simulink library "tinbot"  (R2016a)
settings: Solver=ode45  StartTime=0.0  StopTime=10.0  RelTol=1e-3
libraries: tinbot x23, simulink x4
settings Model: Creator=maximilian  LastModifiedBy=maximilian
settings DataIOCC: LimitDataPoints=on
settings DebuggingCC: AllowSymbolicDim=off

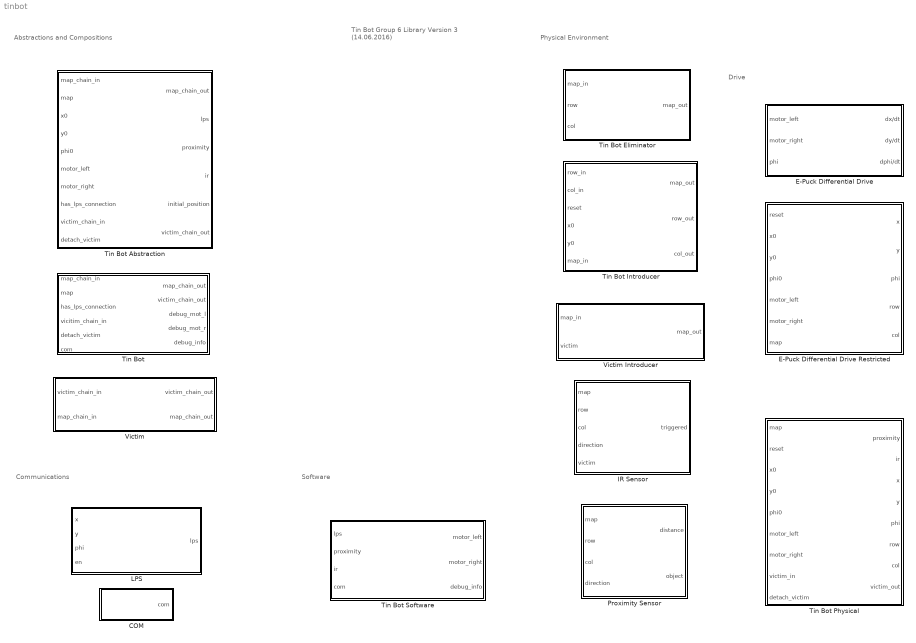
== system tinbot ==
  note: Abstractions and Compositions
  note: Tin Bot
      | Group 6
      |
      | Library
      | Version 3
      | (14.06.2016)
  note: Communications
  note: Physical Environment
  note: Software
  note: Drive
  COM : Subsystem
      mask Display: fprintf('COM')
  E-Puck Differential Drive : Subsystem  TreatAsAtomicUnit=on
      mask Display: fprintf('E-Puck\nDifferential Drive')
  E-Puck Differential Drive Restricted : Subsystem
      mask Display: fprintf('E-Puck\nDifferential Drive\n(restricted)')
  IR Sensor : Subsystem
      mask Display: fprintf('IR Sensor')
  LPS : Subsystem
      mask Display: fprintf('LPS')
  Proximity Sensor : Subsystem
      mask Display: fprintf('Proximity Sensor')
  Tin Bot : Subsystem  mask{x0=100, y0=100, phi0=0}
      mask Display: fprintf('Tin Bot')
  Tin Bot Abstraction : Subsystem
      mask Display: fprintf('Tin Bot\n(abstract)')
  Tin Bot Eliminator : Subsystem
      mask Display: fprintf('Tin Bot\nEliminator')
  Tin Bot Introducer : Subsystem
      mask Display: fprintf('Tin Bot\nIntroducer')
  Tin Bot Physical : Subsystem
      mask Display: fprintf('Tin Bot\nPhysical\n(with motor delay)')
  Tin Bot Software : Subsystem
      mask Display: fprintf('Tin Bot\nSoftware');
  Victim : Subsystem  mask{x0=100, y0=100}
      mask Display: fprintf('Victim')
  Victim Introducer : Subsystem
      mask Display: fprintf('Victim\nIntroducer')

== system tinbot/COM ==
  Chart : Stateflow chart
  com : Outport
  wires:
  Chart/1(com) -> com/1

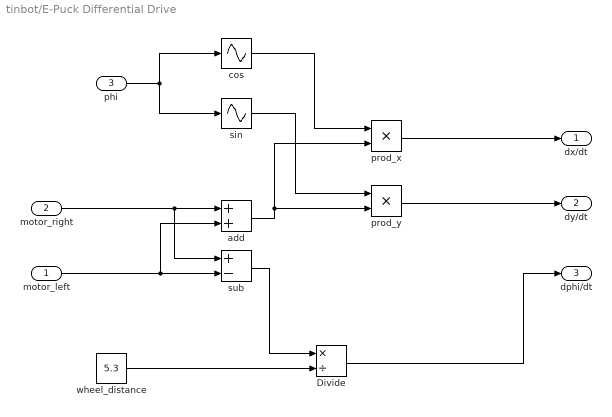
== system tinbot/E-Puck Differential Drive ==
  motor_left : Inport
  motor_right : Inport  Port=2
  phi : Inport  Port=3
  Divide : Product  Inputs=*/
  add : Sum
  cos : Sin  TimeSource=Use external signal  Amplitude=0.5  Phase=pi/2  SampleTime=0
  prod_x : Product
  prod_y : Product
  "sin " : Sin  TimeSource=Use external signal  Amplitude=0.5  SampleTime=0
  sub : Sum  Inputs=+-
  wheel_distance : Constant  Value=5.3
  dx/dt : Outport
  dy/dt : Outport  Port=2
  dphi/dt : Outport  Port=3
  wires:
  motor_left/1 -> sub/2, add/2
  motor_right/1 -> sub/1, add/1
  sub/1 -> Divide/1
  wheel_distance/1 -> Divide/2
  Divide/1 -> dphi/dt/1
  phi/1 -> "sin "/1, cos/1
  add/1 -> prod_x/2, prod_y/2
  "sin "/1 -> prod_y/1
  prod_y/1 -> dy/dt/1
  cos/1 -> prod_x/1
  prod_x/1 -> dx/dt/1

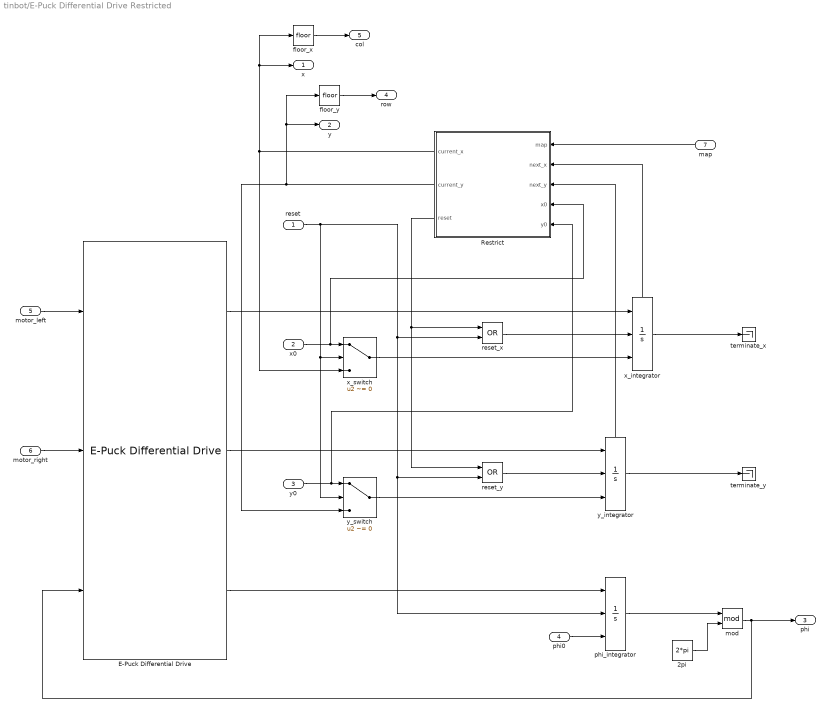
== system tinbot/E-Puck Differential Drive Restricted ==
  reset : Inport
  x0 : Inport  Port=2
  y0 : Inport  Port=3
  phi0 : Inport  Port=4
  motor_left : Inport  Port=5
  motor_right : Inport  Port=6
  map : Inport  Port=7
  2pi : Constant  Value=2*pi
  E-Puck Differential Drive : tinbot/E-Puck Differential Drive  SystemSampleTime=-1
  Restrict : Stateflow chart  TreatAsAtomicUnit=on
  floor_x : Rounding
  floor_y : Rounding
  mod : Math  Operator=mod  SaturateOnIntegerOverflow=on
  phi_integrator : Integrator  ExternalReset=rising  InitialConditionSource=external
  reset_x : Logic  Operator=OR  AllPortsSameDT=off  OutDataTypeStr=boolean
  reset_y : Logic  Operator=OR  AllPortsSameDT=off  OutDataTypeStr=boolean
  terminate_x : Terminator
  terminate_y : Terminator
  x_integrator : Integrator  ExternalReset=rising  InitialConditionSource=external  ShowStatePort=on
  x_switch : Switch  Criteria=u2 ~= 0
  y_integrator : Integrator  ExternalReset=rising  InitialConditionSource=external  ShowStatePort=on
  y_switch : Switch  Criteria=u2 ~= 0
  "x " : Outport
  y : Outport  Port=2
  "phi " : Outport  Port=3
  row : Outport  Port=4
  col : Outport  Port=5
  wires:
  E-Puck Differential Drive/1 -> x_integrator/1
  E-Puck Differential Drive/2 -> y_integrator/1
  E-Puck Differential Drive/3 -> phi_integrator/1
  phi_integrator/1 -> mod/1
  motor_left/1 -> E-Puck Differential Drive/1
  motor_right/1 -> E-Puck Differential Drive/2
  reset_x/1 -> x_integrator/2
  Restrict/3(reset) -> reset_y/1, reset_x/1
  reset_y/1 -> y_integrator/2
  x_switch/1 -> x_integrator/3
  reset/1 -> phi_integrator/2, reset_y/2, reset_x/2, x_switch/2, y_switch/2
  y_switch/1 -> y_integrator/3
  x0/1 -> Restrict/4(x0), x_switch/1
  x_integrator/State -> Restrict/2(next_x)
  y_integrator/State -> Restrict/3(next_y)
  phi0/1 -> phi_integrator/3
  y0/1 -> Restrict/5(y0), y_switch/1
  map/1 -> Restrict/1(map)
  floor_x/1 -> col/1
  Restrict/1(current_x) -> floor_x/1, "x "/1, x_switch/3
  floor_y/1 -> row/1
  Restrict/2(current_y) -> y/1, floor_y/1, y_switch/3
  x_integrator/1 -> terminate_x/1
  y_integrator/1 -> terminate_y/1
  mod/1 -> E-Puck Differential Drive/3, "phi "/1
  2pi/1 -> mod/2

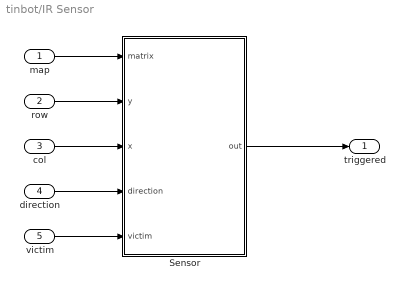
== system tinbot/IR Sensor ==
  map : Inport
  row : Inport  Port=2
  col : Inport  Port=3
  direction : Inport  Port=4
  victim : Inport  Port=5
  Sensor : MATLAB Function  TreatAsAtomicUnit=on
  triggered : Outport  OutDataTypeStr=double
  wires:
  map/1 -> Sensor/1(matrix)
  col/1 -> Sensor/3(x)
  row/1 -> Sensor/2(y)
  direction/1 -> Sensor/4(direction)
  Sensor/1(out) -> triggered/1
  victim/1 -> Sensor/5(victim)

== system tinbot/LPS ==
  x : Inport
  y : Inport  Port=2
  phi : Inport  Port=3
  en : Inport  Port=4
  Chart : Stateflow chart
  lps : Outport
  wires:
  x/1 -> Chart/1(x)
  y/1 -> Chart/2(y)
  phi/1 -> Chart/3(phi)
  en/1 -> Chart/4(en)
  Chart/1(lps) -> lps/1

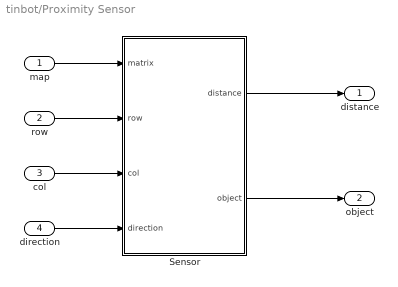
== system tinbot/Proximity Sensor ==
  map : Inport
  row : Inport  Port=2
  col : Inport  Port=3
  direction : Inport  Port=4
  Sensor : MATLAB Function  TreatAsAtomicUnit=on
  distance : Outport
  object : Outport  Port=2
  wires:
  map/1 -> Sensor/1(matrix)
  col/1 -> Sensor/3(col)
  row/1 -> Sensor/2(row)
  direction/1 -> Sensor/4(direction)
  Sensor/1(distance) -> distance/1
  Sensor/2(object) -> object/1

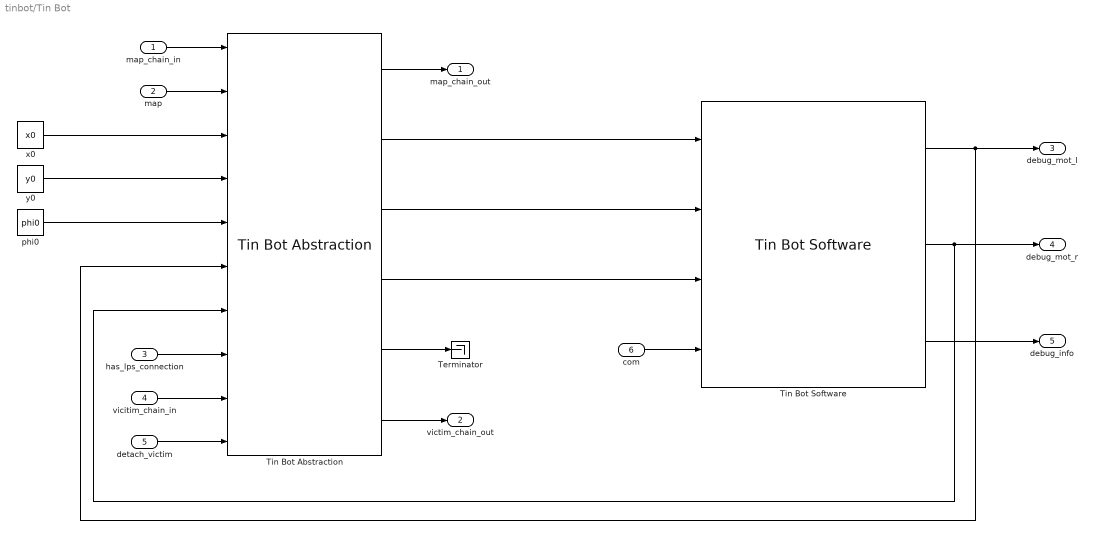
== system tinbot/Tin Bot ==
  map_chain_in : Inport
  map : Inport  Port=2
  has_lps_connection : Inport  Port=3
  vicitim_chain_in : Inport  Port=4
  detach_victim : Inport  Port=5
  com : Inport  Port=6
  Terminator : Terminator
  Tin Bot Abstraction : tinbot/Tin Bot Abstraction  SystemSampleTime=-1
  Tin Bot Software : tinbot/Tin Bot Software  SystemSampleTime=-1
  phi0 : Constant  Value=phi0
  x0 : Constant  Value=x0
  y0 : Constant  Value=y0
  map_chain_out : Outport
  victim_chain_out : Outport  Port=2
  debug_mot_l : Outport  Port=3
  debug_mot_r : Outport  Port=4
  debug_info : Outport  Port=5
  wires:
  map/1 -> Tin Bot Abstraction/2
  map_chain_in/1 -> Tin Bot Abstraction/1
  Tin Bot Abstraction/1 -> map_chain_out/1
  x0/1 -> Tin Bot Abstraction/3
  y0/1 -> Tin Bot Abstraction/4
  phi0/1 -> Tin Bot Abstraction/5
  has_lps_connection/1 -> Tin Bot Abstraction/8
  Tin Bot Software/2 -> Tin Bot Abstraction/7, debug_mot_r/1
  vicitim_chain_in/1 -> Tin Bot Abstraction/9
  Tin Bot Abstraction/6 -> victim_chain_out/1
  detach_victim/1 -> Tin Bot Abstraction/10
  Tin Bot Abstraction/5 -> Terminator/1
  Tin Bot Abstraction/4 -> Tin Bot Software/3
  Tin Bot Abstraction/3 -> Tin Bot Software/2
  Tin Bot Abstraction/2 -> Tin Bot Software/1
  Tin Bot Software/1 -> Tin Bot Abstraction/6, debug_mot_l/1
  Tin Bot Software/3 -> debug_info/1
  com/1 -> Tin Bot Software/4

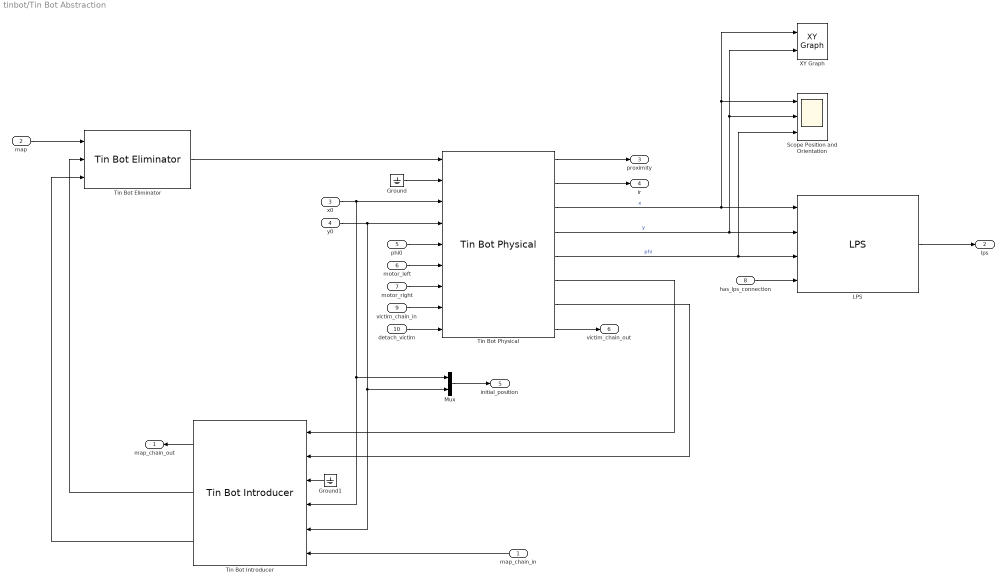
== system tinbot/Tin Bot Abstraction ==
  map_chain_in : Inport
  map : Inport  Port=2
  x0 : Inport  Port=3
  y0 : Inport  Port=4
  phi0 : Inport  Port=5
  motor_left : Inport  Port=6
  motor_right : Inport  Port=7
  has_lps_connection : Inport  Port=8
  victim_chain_in : Inport  Port=9
  detach_victim : Inport  Port=10
  Ground : Ground
  Ground1 : Ground
  LPS : tinbot/LPS  SystemSampleTime=-1
  Mux : Mux  Inputs=2
  Scope Position and Orientation : Scope  NumInputPorts=3
  Tin Bot Eliminator : tinbot/Tin Bot Eliminator  SystemSampleTime=-1
  Tin Bot Introducer : tinbot/Tin Bot Introducer  SystemSampleTime=-1
  Tin Bot Physical : tinbot/Tin Bot Physical  SystemSampleTime=-1
  XY Graph : simulink/Sinks/XY Graph  xmin=1  xmax=200  ymin=1  ymax=200  st=-1
  map_chain_out : Outport
  lps : Outport  Port=2
  proximity : Outport  Port=3
  ir : Outport  Port=4
  initial_position : Outport  Port=5
  victim_chain_out : Outport  Port=6
  wires:
  Tin Bot Eliminator/1 -> Tin Bot Physical/1
  Tin Bot Physical/6 -> Tin Bot Introducer/1
  Tin Bot Physical/7 -> Tin Bot Introducer/2
  Tin Bot Introducer/3 -> Tin Bot Eliminator/3
  Tin Bot Introducer/2 -> Tin Bot Eliminator/2
  map_chain_in/1 -> Tin Bot Introducer/6
  Tin Bot Introducer/1 -> map_chain_out/1
  map/1 -> Tin Bot Eliminator/1
  y0/1 -> Tin Bot Physical/4, Mux/2, Tin Bot Introducer/5
  Ground/1 -> Tin Bot Physical/2
  Ground1/1 -> Tin Bot Introducer/3
  phi0/1 -> Tin Bot Physical/5
  motor_left/1 -> Tin Bot Physical/6
  motor_right/1 -> Tin Bot Physical/7
  Tin Bot Physical/4 -> XY Graph/2, Scope Position and Orientation/2, LPS/2  "y"
  Tin Bot Physical/5 -> Scope Position and Orientation/3, LPS/3  "phi"
  has_lps_connection/1 -> LPS/4
  LPS/1 -> lps/1
  Tin Bot Physical/1 -> proximity/1
  Tin Bot Physical/2 -> ir/1
  Mux/1 -> initial_position/1
  Tin Bot Physical/3 -> XY Graph/1, Scope Position and Orientation/1, LPS/1  "x"
  x0/1 -> Tin Bot Physical/3, Tin Bot Introducer/4, Mux/1
  victim_chain_in/1 -> Tin Bot Physical/8
  Tin Bot Physical/8 -> victim_chain_out/1
  detach_victim/1 -> Tin Bot Physical/9

== system tinbot/Tin Bot Eliminator ==
  map_in : Inport  PortDimensions=[200 200]
  row : Inport  Port=2
  col : Inport  Port=3
  Tin Bot Eliminator : MATLAB Function  TreatAsAtomicUnit=on
  map_out : Outport  PortDimensions=[200 200]
  wires:
  row/1 -> Tin Bot Eliminator/2(row)
  col/1 -> Tin Bot Eliminator/3(col)
  Tin Bot Eliminator/1(map_out) -> map_out/1
  map_in/1 -> Tin Bot Eliminator/1(map_in)

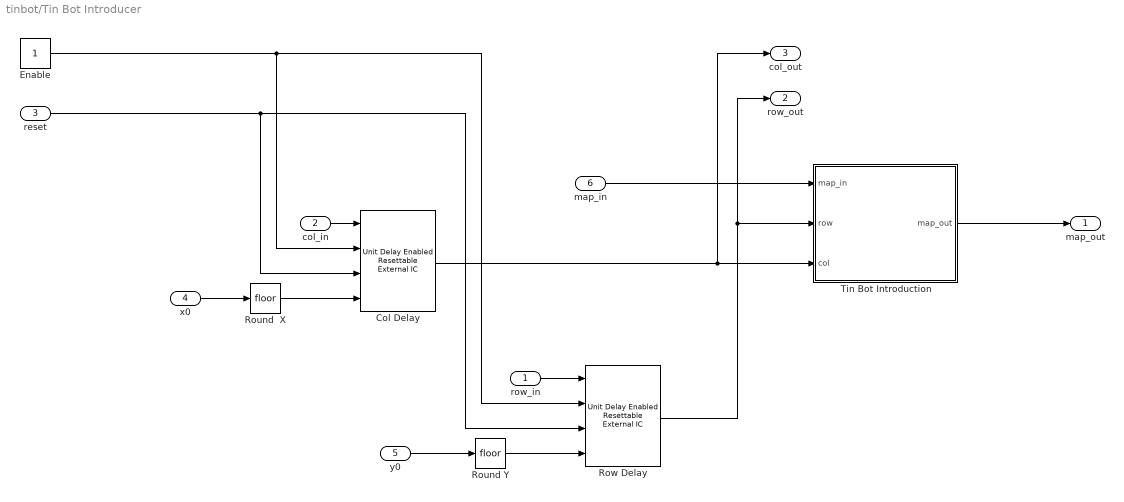
== system tinbot/Tin Bot Introducer ==
  row_in : Inport  Interpolate=off
  col_in : Inport  Port=2  Interpolate=off
  reset : Inport  Port=3
  x0 : Inport  Port=4
  y0 : Inport  Port=5
  map_in : Inport  Port=6  PortDimensions=[200 200]  Interpolate=off
  Col Delay : simulink/Additional Math & Discrete/Additional Discrete/Unit Delay Enabled Resettable External IC  tsamp=-1
  Enable : Constant
  Round  X : Rounding
  Round Y : Rounding
  Row Delay : simulink/Additional Math & Discrete/Additional Discrete/Unit Delay Enabled Resettable External IC  tsamp=-1
  Tin Bot Introduction : MATLAB Function  TreatAsAtomicUnit=on
  map_out : Outport  PortDimensions=[200 200]
  row_out : Outport  Port=2
  col_out : Outport  Port=3
  wires:
  reset/1 -> Row Delay/3, Col Delay/3
  y0/1 -> Round Y/1
  Round Y/1 -> Row Delay/4
  Round  X/1 -> Col Delay/4
  x0/1 -> Round  X/1
  Enable/1 -> Row Delay/2, Col Delay/2
  col_in/1 -> Col Delay/1
  row_in/1 -> Row Delay/1
  Col Delay/1 -> col_out/1, Tin Bot Introduction/3(col)
  Row Delay/1 -> row_out/1, Tin Bot Introduction/2(row)
  map_in/1 -> Tin Bot Introduction/1(map_in)
  Tin Bot Introduction/1(map_out) -> map_out/1

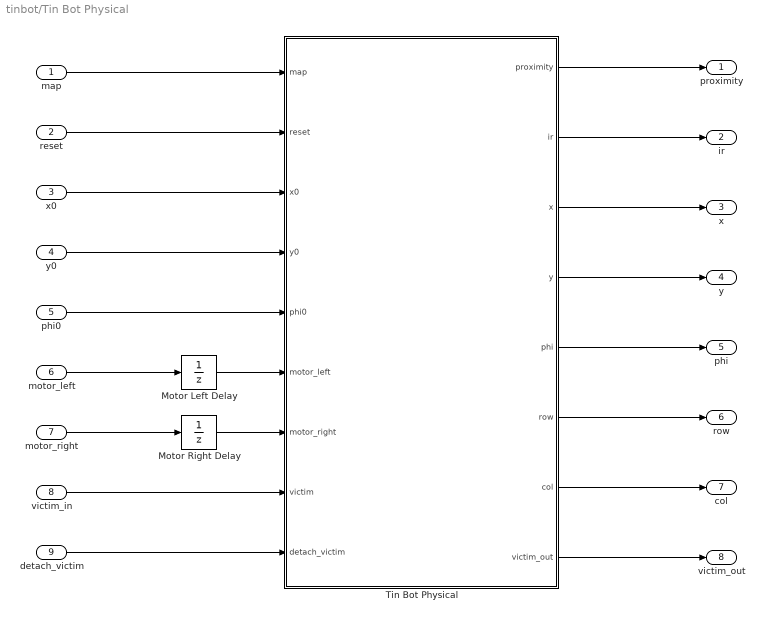
== system tinbot/Tin Bot Physical ==
  map : Inport
  reset : Inport  Port=2
  x0 : Inport  Port=3
  y0 : Inport  Port=4
  phi0 : Inport  Port=5
  motor_left : Inport  Port=6
  motor_right : Inport  Port=7
  victim_in : Inport  Port=8
  detach_victim : Inport  Port=9
  Motor Left Delay : UnitDelay  SampleTime=-1
  Motor Right Delay : UnitDelay  SampleTime=-1
  Tin Bot Physical : Subsystem  TreatAsAtomicUnit=on
  proximity : Outport
  ir : Outport  Port=2
  x : Outport  Port=3
  y : Outport  Port=4
  phi : Outport  Port=5
  row : Outport  Port=6
  col : Outport  Port=7
  victim_out : Outport  Port=8
  wires:
  Motor Left Delay/1 -> Tin Bot Physical/6(motor_left)
  Motor Right Delay/1 -> Tin Bot Physical/7(motor_right)
  map/1 -> Tin Bot Physical/1(map)
  reset/1 -> Tin Bot Physical/2(reset)
  x0/1 -> Tin Bot Physical/3(x0)
  y0/1 -> Tin Bot Physical/4(y0)
  phi0/1 -> Tin Bot Physical/5(phi0)
  motor_left/1 -> Motor Left Delay/1
  motor_right/1 -> Motor Right Delay/1
  Tin Bot Physical/1(proximity) -> proximity/1
  Tin Bot Physical/2(ir) -> ir/1
  Tin Bot Physical/3(x) -> x/1
  Tin Bot Physical/4(y) -> y/1
  Tin Bot Physical/5(phi) -> phi/1
  Tin Bot Physical/6(row) -> row/1
  Tin Bot Physical/7(col) -> col/1
  victim_in/1 -> Tin Bot Physical/8(victim)
  Tin Bot Physical/8(victim_out) -> victim_out/1
  detach_victim/1 -> Tin Bot Physical/9(detach_victim)

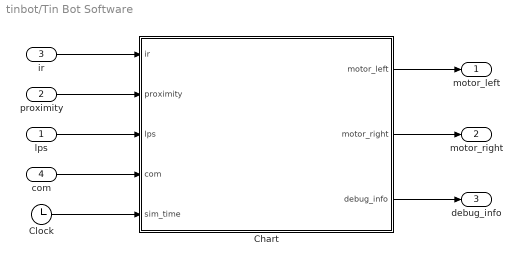
== system tinbot/Tin Bot Software ==
  lps : Inport
  proximity : Inport  Port=2
  ir : Inport  Port=3
  com : Inport  Port=4
  Chart : Stateflow chart
  Clock : Clock
  motor_left : Outport
  motor_right : Outport  Port=2
  debug_info : Outport  Port=3
  wires:
  lps/1 -> Chart/3(lps)
  proximity/1 -> Chart/2(proximity)
  ir/1 -> Chart/1(ir)
  Chart/1(motor_left) -> motor_left/1
  Chart/2(motor_right) -> motor_right/1
  Clock/1 -> Chart/5(sim_time)
  Chart/3(debug_info) -> debug_info/1
  com/1 -> Chart/4(com)

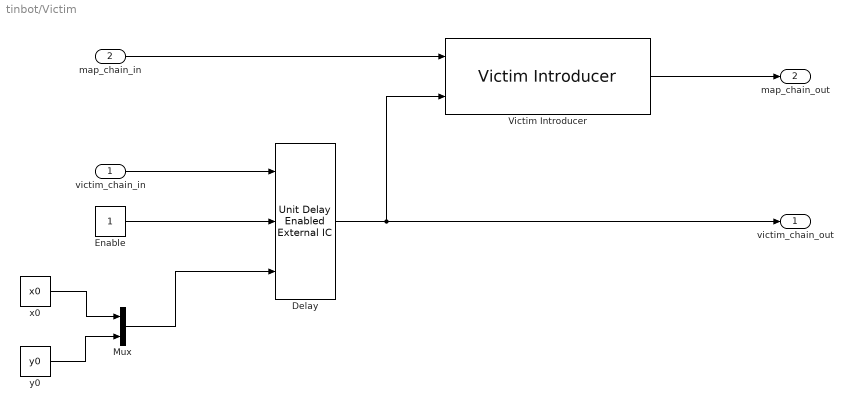
== system tinbot/Victim ==
  victim_chain_in : Inport
  map_chain_in : Inport  Port=2
  Delay : simulink/Additional Math & Discrete/Additional Discrete/Unit Delay Enabled External IC  tsamp=-1
  Enable : Constant
  Mux : Mux  Inputs=2
  Victim Introducer : tinbot/Victim Introducer  SystemSampleTime=-1
  x0 : Constant  Value=x0
  y0 : Constant  Value=y0
  victim_chain_out : Outport
  map_chain_out : Outport  Port=2
  wires:
  victim_chain_in/1 -> Delay/1
  Delay/1 -> Victim Introducer/2, victim_chain_out/1
  Enable/1 -> Delay/2
  Mux/1 -> Delay/3
  x0/1 -> Mux/1
  y0/1 -> Mux/2
  map_chain_in/1 -> Victim Introducer/1
  Victim Introducer/1 -> map_chain_out/1

== system tinbot/Victim Introducer ==
  map_in : Inport  PortDimensions=[200 200]  Interpolate=off
  victim : Inport  Port=2
  Victim Introduction : MATLAB Function  TreatAsAtomicUnit=on
  map_out : Outport  PortDimensions=[200 200]
  wires:
  map_in/1 -> Victim Introduction/1(map_in)
  Victim Introduction/1(map_out) -> map_out/1
  victim/1 -> Victim Introduction/2(victim)

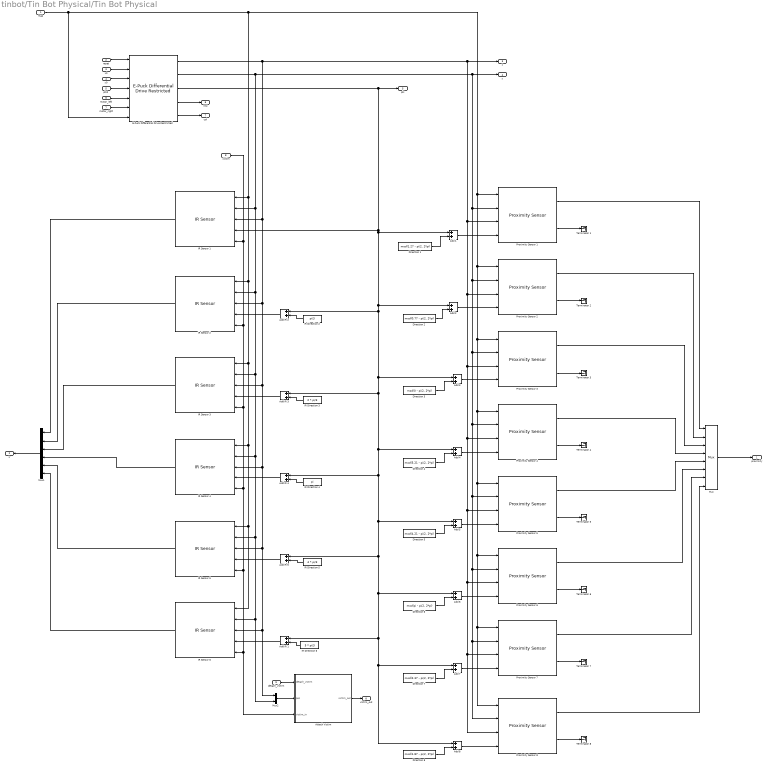
== system tinbot/Tin Bot Physical/Tin Bot Physical ==
  map : Inport
  reset : Inport  Port=2
  x0 : Inport  Port=3
  y0 : Inport  Port=4
  phi0 : Inport  Port=5
  motor_left : Inport  Port=6
  motor_right : Inport  Port=7
  victim : Inport  Port=8
  detach_victim : Inport  Port=9
  Add {1..8} (8 alike) : Sum
  Add IR {1..5} (5 alike) : Sum
  Attach Victim : Stateflow chart  TreatAsAtomicUnit=on
  Direction 1 : Constant  Value=mod(1.27 - pi/2, 2*pi)
  Direction 2 : Constant  Value=mod(0.77 - pi/2, 2*pi)
  Direction 3 : Constant  Value=mod(0 - pi/2, 2*pi)
  Direction 4 : Constant  Value=mod(5.21 - pi/2, 2*pi)
  Direction 5 : Constant  Value=mod(4.21 - pi/2, 2*pi)
  Direction 6 : Constant  Value=mod(pi - pi/2, 2*pi)
  Direction 7 : Constant  Value=mod(2.37 - pi/2, 2*pi)
  Direction 8 : Constant  Value=mod(1.87 - pi/2, 2*pi)
  E-Puck Differential Drive Restricted : tinbot/E-Puck Differential Drive Restricted  SystemSampleTime=-1
  IR Direction 2 : Constant  Value=pi/3
  IR Direction 3 : Constant  Value=2 * pi/3
  IR Direction 4 : Constant  Value=pi
  IR Direction 5 : Constant  Value=4 * pi/3
  IR Direction 6 : Constant  Value=5 * pi/3
  IR Sensor {1..6} (6 alike) : tinbot/IR Sensor  SystemSampleTime=-1
  Mux : Mux  Inputs=8
  Mux1 : Mux  Inputs=6
  Mux2 : Mux  Inputs=2
  Proximity Sensor {1..8} (8 alike) : tinbot/Proximity Sensor  SystemSampleTime=-1
  Terminator {1..8} (8 alike) : Terminator
  proximity : Outport  PortDimensions=8
  ir : Outport  Port=2  PortDimensions=6
  x : Outport  Port=3
  y : Outport  Port=4
  phi : Outport  Port=5
  row : Outport  Port=6
  col : Outport  Port=7
  victim_out : Outport  Port=8
  wires:
  map/1 -> E-Puck Differential Drive Restricted/7, Proximity Sensor 1/1, Proximity Sensor 2/1, Proximity Sensor 3/1, Proximity Sensor 4/1, Proximity Sensor 5/1, Proximity Sensor 6/1, Proximity Sensor 8/1, Proximity Sensor 7/1, IR Sensor 1/1, IR Sensor 2/1, IR Sensor 3/1, IR Sensor 4/1, IR Sensor 6/1, IR Sensor 5/1
  Add 1/1 -> Proximity Sensor 1/4
  Direction 1/1 -> Add 1/2
  Add 2/1 -> Proximity Sensor 2/4
  Direction 2/1 -> Add 2/2
  Add 3/1 -> Proximity Sensor 3/4
  Direction 3/1 -> Add 3/2
  Add 4/1 -> Proximity Sensor 4/4
  Direction 4/1 -> Add 4/2
  Add 5/1 -> Proximity Sensor 5/4
  Direction 5/1 -> Add 5/2
  Add 6/1 -> Proximity Sensor 6/4
  Direction 6/1 -> Add 6/2
  Add 7/1 -> Proximity Sensor 7/4
  Direction 7/1 -> Add 7/2
  Add 8/1 -> Proximity Sensor 8/4
  Direction 8/1 -> Add 8/2
  E-Puck Differential Drive Restricted/4 -> row/1
  Proximity Sensor 1/1 -> Mux/1
  Proximity Sensor 2/1 -> Mux/2
  Proximity Sensor 3/1 -> Mux/3
  Proximity Sensor 4/1 -> Mux/4
  Proximity Sensor 5/1 -> Mux/5
  Proximity Sensor 6/1 -> Mux/6
  Proximity Sensor 7/1 -> Mux/7
  Proximity Sensor 8/1 -> Mux/8
  Mux/1 -> proximity/1
  E-Puck Differential Drive Restricted/3 -> phi/1, Add 8/1, Add 7/1, Add IR 1/1, Add 6/1, Add IR 5/1, Add 5/1, Add IR 4/1, Add 4/1, Add IR 3/1, Add 3/1, Add IR 2/1, Add 2/1, Add 1/1, IR Sensor 1/4
  Add IR 2/1 -> IR Sensor 2/4
  IR Direction 2/1 -> Add IR 2/2
  IR Direction 3/1 -> Add IR 3/2
  Add IR 3/1 -> IR Sensor 3/4
  IR Direction 4/1 -> Add IR 4/2
  Add IR 4/1 -> IR Sensor 4/4
  Add IR 5/1 -> IR Sensor 5/4
  IR Direction 5/1 -> Add IR 5/2
  Add IR 1/1 -> IR Sensor 6/4
  IR Direction 6/1 -> Add IR 1/2
  IR Sensor 1/1 -> Mux1/1
  IR Sensor 2/1 -> Mux1/2
  IR Sensor 3/1 -> Mux1/3
  IR Sensor 4/1 -> Mux1/4
  IR Sensor 5/1 -> Mux1/5
  Mux1/1 -> ir/1
  Proximity Sensor 5/2 -> Terminator 5/1
  Proximity Sensor 6/2 -> Terminator 6/1
  Proximity Sensor 4/2 -> Terminator 4/1
  Proximity Sensor 3/2 -> Terminator 3/1
  Proximity Sensor 2/2 -> Terminator 2/1
  Proximity Sensor 1/2 -> Terminator 1/1
  Proximity Sensor 7/2 -> Terminator 7/1
  Proximity Sensor 8/2 -> Terminator 8/1
  E-Puck Differential Drive Restricted/5 -> col/1
  reset/1 -> E-Puck Differential Drive Restricted/1
  x0/1 -> E-Puck Differential Drive Restricted/2
  y0/1 -> E-Puck Differential Drive Restricted/3
  phi0/1 -> E-Puck Differential Drive Restricted/4
  motor_left/1 -> E-Puck Differential Drive Restricted/5
  motor_right/1 -> E-Puck Differential Drive Restricted/6
  IR Sensor 6/1 -> Mux1/6
  E-Puck Differential Drive Restricted/2 -> Proximity Sensor 1/2, Proximity Sensor 2/2, Proximity Sensor 3/2, Proximity Sensor 4/2, Proximity Sensor 5/2, Proximity Sensor 6/2, Proximity Sensor 8/2, Proximity Sensor 7/2, y/1, IR Sensor 1/2, IR Sensor 2/2, IR Sensor 3/2, IR Sensor 4/2, Mux2/2, IR Sensor 6/2, IR Sensor 5/2
  E-Puck Differential Drive Restricted/1 -> IR Sensor 1/3, IR Sensor 2/3, IR Sensor 3/3, IR Sensor 4/3, Mux2/1, IR Sensor 6/3, IR Sensor 5/3, Proximity Sensor 1/3, Proximity Sensor 2/3, Proximity Sensor 3/3, Proximity Sensor 4/3, Proximity Sensor 5/3, Proximity Sensor 6/3, Proximity Sensor 8/3, Proximity Sensor 7/3, x/1
  victim/1 -> Attach Victim/3(victim_in), IR Sensor 6/5, IR Sensor 5/5, IR Sensor 4/5, IR Sensor 3/5, IR Sensor 2/5, IR Sensor 1/5
  Mux2/1 -> Attach Victim/2(pos)
  detach_victim/1 -> Attach Victim/1(detach_victim)
  Attach Victim/1(victim_out) -> victim_out/1

== matlab function tinbot/Tin Bot Eliminator/Tin Bot Eliminator ==
  data: map_in input; map_out output; row input; col input
function map_out = eliminate(map_in, row, col)
    map_in(row-2, col) = 0;
    
    map_in(row-1, col-1) = 0;
    map_in(row-1, col) = 0;
    map_in(row-1, col+1) = 0;
    
    map_in(row, col+2) = 0;
    map_in(row, col+1) = 0;
    map_in(row, col) = 0;
    map_in(row, col-1) = 0;
    map_in(row, col-2) = 0;
    
    map_in(row+1, col-1) = 0;
    map_in(row+1, col) = 0;
    map_in(row+1, col+1) = 0;
    
    map_in(row+2, col) = 0;
    
    map_out = map_in;

== matlab function tinbot/Tin Bot Introducer/Tin Bot Introduction ==
  data: map_in input; map_out output; row input; col input
function map_out = introduce(map_in, row, col)
    map_in(row-2, col) = 3;
    
    map_in(row-1, col-1) = 3;
    map_in(row-1, col) = 3;
    map_in(row-1, col+1) = 3;
    
    map_in(row, col+2) = 3;
    map_in(row, col+1) = 3;
    map_in(row, col) = 3;
    map_in(row, col-1) = 3;
    map_in(row, col-2) = 3;
    
    map_in(row+1, col-1) = 3;
    map_in(row+1, col) = 3;
    map_in(row+1, col+1) = 3;
    
    map_in(row+2, col) = 3;
    
    map_out = map_in;

== stateflow chart tinbot/E-Puck Differential Drive Restricted/Restrict ==
  state Start
  state Reset
  (default) -> Start : {
      | 	current_x = x0; current_y = y0; reset = 0;
      | 	x = current_x; y = current_y;
      | 	col = floor(x) + 1; row = floor(y) + 1
      | }
  Start -> Start [order 2] : {
      | 	x = next_x; y = next_y;
      | 	col = floor(y); row = floor(x) ;
      | 	current_x = x;
      | 	current_y = y;
      | }
  Reset -> Start : {reset = 0;}
  Start -> Reset [order 1] : [(floor(next_y) ~= row || floor(next_x) ~= col) && (map(floor(next_y)-2, floor(next_x)) ~= 0 || map(floor(next_y)+2, floor(next_x)) ~= 0 || map(floor(next_y), floor(next_x)-2) ~= 0 || map(floor(next_y), floor(next_x)+2) ~= 0 || map(floor(next_y)+1, floor(next_x)+1) ~= 0 || map(floor(next_y)+1, floor(next_x)-1) ~= 0 || map(floor(next_y)-1, floor(next_x)+1) ~= 0 || map(floor(next_y)-1, floor(next_x)-1) ~= 0)]{
      | 	reset = 1;
      | 	current_x = x;
      | 	current_y = y;
      | }
  data: map input; next_x input; next_y input; current_x output =0; current_y output =0; reset output =0; x local; y local; x0 input; y0 input; col local; row local

== matlab function tinbot/Proximity Sensor/Sensor ==
  data: matrix input; row input; col input; distance output; direction input; object output
function [distance, object] = raycast(matrix, row, col, direction)
    % A better value can be obtained at:
    % http://www.e-puck.org/index.php?option=com_content&view=article&id=22&Itemid=13
    max_distance = 12.8;
    [distance, object] = TinUtils.raycast_polymorphic(matrix, row, col, direction, max_distance);
end

== matlab function tinbot/IR Sensor/Sensor ==
  data: matrix input; y input; x input; out output; direction input; victim input
function out  = raycast(matrix, y, x, direction, victim)
    out = 0;
    victim_direction = atan2(victim(2) - y, victim(1) - x);
    delta = abs(mod(victim_direction - direction + pi, 2 * pi) - pi);
    if delta < deg2rad(40);
        [~, object] = TinUtils.raycast_polymorphic(matrix, y, x, victim_direction, 400);
        if (object == 2)
            out =1;
        end
    end
end

== stateflow chart tinbot/LPS/Chart ==
  state Init
  state Start
  state Send
  (default) -> Init : {
      | 	lps = [x; y; phi];
      | }
  Init -> Start : {
      | 	lps = [-1; -1; -1];
      | }
  Send -> Start : {
      | 	lps = [-1; -1; -1];
      | }
  Start -> Send : [after(2, sec) && en == 1] {
      | 	lps = [x; y; phi];
      | }
  data: x input; y input; phi input; en input; lps output

== stateflow chart tinbot/Tin Bot Software/Chart ==
  state Start_
    entry:
    tinbot = matlab_create_bot();
    during:
    matlab_select_bot(tinbot, com);
    matlab_update_proximity(proximity);
    matlab_update_ir(ir);
    matlab_update_lps(lps);
    matlab_update_time(sim_time);
    matlab_loop();
    motor_left = matlab_get_motor_left();
    motor_right = matlab_get_motor_right();
    debug_info[0] = matlab_get_debug_info(0);
    debug_info[1] = matlab_get_debug_info(1);
    debug_info[2] = matlab_get_debug_info(2);
    debug_info[3] = matlab_get_debug_info(3);
    debug_info[4] = matlab_get_debug_info(4);
    debug_info[5] = matlab_get_debug_info(5);
    debug_info[6] = matlab_get_debug_info(6);
    debug_info[7] = matlab_get_debug_info(7);
    debug_info[8] = matlab_get_debug_info(8);
    debug_info[9] = matlab_get_debug_info(9);
  (default) -> Start_
  data: ir input size=6; proximity input size=8; motor_left output double; motor_right output double; tinbot local double; lps input size=3; debug_info output double size=10 =zeros(1,10); com input double; sim_time input double

== matlab function tinbot/Victim Introducer/Victim Introduction ==
  data: map_in input; map_out output size=[200 200]; victim input
function map_out = introduce(map_in, victim)
    col = floor(victim(1));
    row = floor(victim(2));
    
    map_in(row-1, col) = 2;

    map_in(row, col+1) = 2;
    map_in(row, col) = 2;
    map_in(row, col-1) = 2;
    
    map_in(row+1, col) = 2;
    
    map_out = map_in;

== stateflow chart tinbot/Tin Bot Physical/Tin Bot Physical/Attach Victim ==
  state Attached
    entry, during:
    direction = atan2(victim_in(2) - pos(2), victim_in(1) - pos(1));
    victim_out = pos + [(cos(direction) * TinUtils.pickup_distance); (sin(direction) * TinUtils.pickup_distance)];
  state Start
    entry, during:
    victim_out = victim_in;
  state Detaching
    entry, during:
    victim_out = victim_in;
  (default) -> Start
  Start -> Attached : [norm(victim_in - pos) <= TinUtils.pickup_distance]
  Attached -> Detaching : [detach_victim > 0]
  Detaching -> Start : [norm(victim_in - pos) > TinUtils.pickup_distance]
  data: detach_victim input; pos input; victim_in input; victim_out output; direction local

== stateflow chart tinbot/COM/Chart ==
  state Start_
    entry:
    com = matlab_create_com();
  (default) -> Start_
  data: com output double
